simulink model "yaw"  (R2020b)
settings: Solver=VariableStepAuto  StartTime=0.0  StopTime=10.0  RelTol=1e-3
settings Model: Creator=User  LastModifiedBy=Matthew

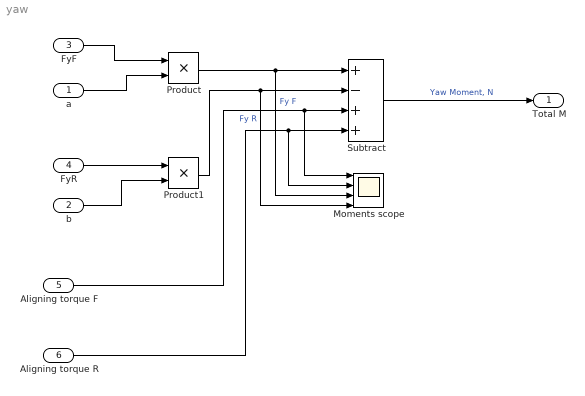
== system yaw ==
  a : Inport
  b : Inport  Port=2
  FyF : Inport  Port=3
  FyR : Inport  Port=4
  Aligning torque F : Inport  Port=5
  Aligning torque R : Inport  Port=6
  Moments scope : Scope  NumInputPorts=4
  Product : Product
  Product1 : Product
  Subtract : Sum  Inputs=+-++
  Total M : Outport
  wires:
  FyF/1 -> Product/1
  a/1 -> Product/2
  FyR/1 -> Product1/1
  b/1 -> Product1/2
  Product1/1 -> Moments scope/4, Subtract/2  "Fy R"
  Product/1 -> Moments scope/3, Subtract/1  "Fy F"
  Subtract/1 -> Total M/1  "Yaw Moment, N"
  Aligning torque F/1 -> Subtract/3, Moments scope/1
  Aligning torque R/1 -> Subtract/4, Moments scope/2
